simulink model "Modelling_of_DifferentialEquations"  (R2017b)
settings: Solver=VariableStepAuto  StartTime=0.0  StopTime=1  RelTol=1e-3
settings Model: Creator=Mahe  LastModifiedBy=Mahe

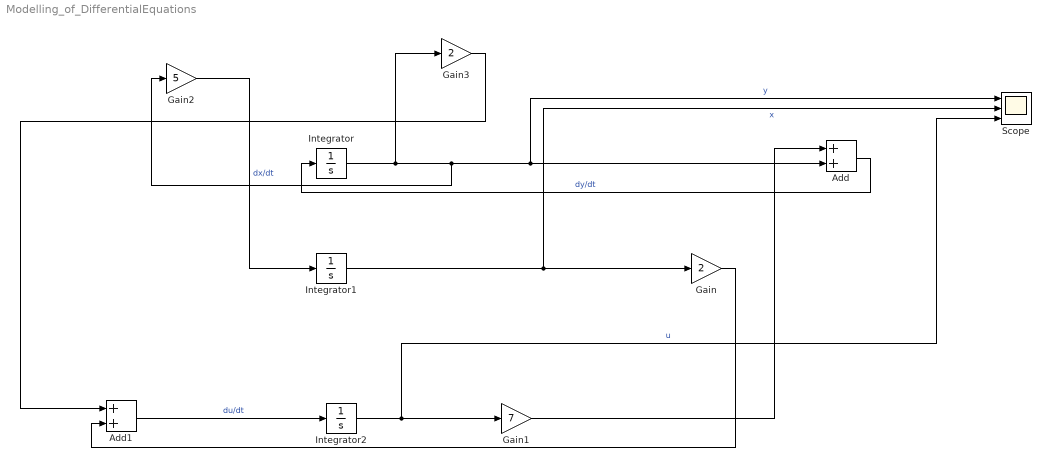
== system Modelling_of_DifferentialEquations ==
  Add : Sum
  Add1 : Sum
  Gain : Gain  Gain=2
  Gain1 : Gain  Gain=7
  Gain2 : Gain  Gain=5
  Gain3 : Gain  Gain=2
  Integrator : Integrator  InitialCondition=1
  Integrator1 : Integrator  InitialCondition=2
  Integrator2 : Integrator
  Scope : Scope  NumInputPorts=3
  wires:
  Integrator/1 -> Gain3/1, Gain2/1, Scope/1, Add/2  "y"
  Integrator1/1 -> Scope/2, Gain/1  "x"
  Integrator2/1 -> Scope/3, Gain1/1  "u"
  Add/1 -> Integrator/1  "dy/dt"
  Gain2/1 -> Integrator1/1  "dx/dt"
  Add1/1 -> Integrator2/1  "du/dt"
  Gain1/1 -> Add/1
  Gain/1 -> Add1/2
  Gain3/1 -> Add1/1
